simulink model "GDFLIB_FilterIIR2_BAM_F16"  (Simulink 8.3)
settings: Solver=ode45  StartTime=0.0  StopTime=10.0  RelTol=1e-3
undefined symbols (not defined in the file): f16A1, f16A2, f16B0, f16B1, f16B2
settings Model: Creator=B17364  LastModifiedBy=B17364
settings OptimizationCC: ExpressionDepthLimit=2147483647
settings DebuggingCC: FcnCallInpInsideContextMsg=UseLocalSettings  StrictBusMsg=Warning

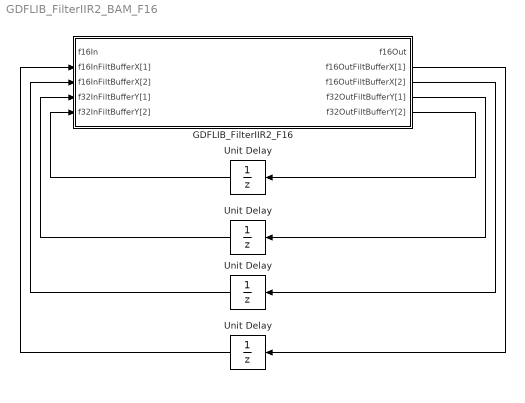
== system GDFLIB_FilterIIR2_BAM_F16 ==
  " Unit Delay" : UnitDelay  SampleTime=-1
  " Unit Delay " : UnitDelay  SampleTime=-1
  GDFLIB_FilterIIR2_F16 : Subsystem  mask(GDFLIB_FilterIIR2){f16B0=f16B0, f16B1=f16B1, f16B2=f16B2, f16A1=f16A1, f16A2=f16A2}
      mask help: Bit accurate model of direct form I second order IIR filter. All parameters as well as input and output are 16bit integers.
      mask init:
      | pos = get_param(gcb, 'Position');width = pos(3) - pos(1); height = pos(4) - pos(2);tX=width/2;tY=height*0.9;
      mask Display: color('black');port_label('input',1,'f16In');port_label('input',2,'f16InFiltBufferX[1]');port_label('input',3,'f16InFiltBufferX[2]');port_label('input',4,'f32InFiltBufferY[1]');port_label('input',5,'f32InFiltBufferY[2]');port_label('output',1,'f16Out');port_label('output',2,'f16OutFiltBufferX[1]');port_label('output',3,'f16OutFiltBufferX[2]');port_label('output',4,'f32OutFiltBufferY[1]');port_label('output',5,'f32OutFiltBufferY[2]');color('black');disp('GDFLIB_FilterIIR2_F16');color('blue');text(tX,tY, 'BAM', 'horizontalAlignment', 'center');
  Unit Delay : UnitDelay  SampleTime=-1
  "Unit Delay " : UnitDelay  SampleTime=-1
  wires:
  GDFLIB_FilterIIR2_F16/2(f16OutFiltBufferX[1]) -> " Unit Delay "/1
  GDFLIB_FilterIIR2_F16/3(f16OutFiltBufferX[2]) -> " Unit Delay"/1
  GDFLIB_FilterIIR2_F16/4(f32OutFiltBufferY[1]) -> "Unit Delay "/1
  GDFLIB_FilterIIR2_F16/5(f32OutFiltBufferY[2]) -> Unit Delay/1
  Unit Delay/1 -> GDFLIB_FilterIIR2_F16/5(f32InFiltBufferY[2])
  "Unit Delay "/1 -> GDFLIB_FilterIIR2_F16/4(f32InFiltBufferY[1])
  " Unit Delay"/1 -> GDFLIB_FilterIIR2_F16/3(f16InFiltBufferX[2])
  " Unit Delay "/1 -> GDFLIB_FilterIIR2_F16/2(f16InFiltBufferX[1])

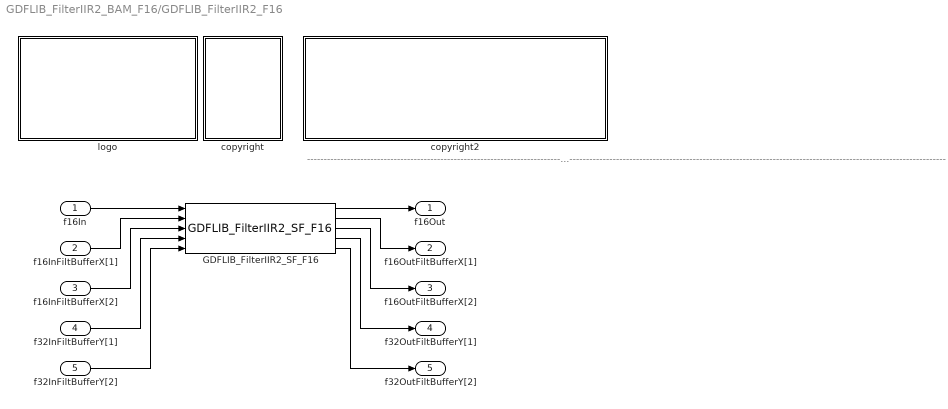
== system GDFLIB_FilterIIR2_BAM_F16/GDFLIB_FilterIIR2_F16 ==
  note: ---------------------------------------------------------------------------------------------------------------------------------------------------------------------------------------------------
  f16In : Inport
  f16InFiltBufferX[1] : Inport  Port=2
  f16InFiltBufferX[2] : Inport  Port=3
  f32InFiltBufferY[1] : Inport  Port=4
  f32InFiltBufferY[2] : Inport  Port=5
  GDFLIB_FilterIIR2_SF_F16 : S-Function  FunctionName=GDFLIB_FilterIIR2_SF_F16  Parameters=f16B0,f16B1,f16B2,f16A1,f16A2  EnableBusSupport=off
  copyright : Subsystem
      mask Display:
      | text(10,90,'FILE:');text(10,75,'DESRIPTION:')
      | text(10,60,'COPYRIGHT:')
      | text(10,45,'VERSION:')
      | text(10,30,'DATE:')
      | text(10,15,'AUTHOR:')
  copyright2 : Subsystem
      mask Display:
      | text(10,90,'GDFLIB_FilterIIR2_BAM_F16.mdl');text(10,75,'Direct form I first order IIR filter.');text(10,60,'Freescale')
      | text(10,45,'0.1');text(10,30,'08-Apr-2014');text(10,15,'');
  logo : Subsystem
      mask Display: image(imread('logo.jpg'))
  f16Out : Outport
  f16OutFiltBufferX[1] : Outport  Port=2
  f16OutFiltBufferX[2] : Outport  Port=3
  f32OutFiltBufferY[1] : Outport  Port=4
  f32OutFiltBufferY[2] : Outport  Port=5
  wires:
  f16In/1 -> GDFLIB_FilterIIR2_SF_F16/1
  GDFLIB_FilterIIR2_SF_F16/1 -> f16Out/1
  GDFLIB_FilterIIR2_SF_F16/2 -> f16OutFiltBufferX[1]/1
  GDFLIB_FilterIIR2_SF_F16/3 -> f16OutFiltBufferX[2]/1
  GDFLIB_FilterIIR2_SF_F16/5 -> f32OutFiltBufferY[2]/1
  GDFLIB_FilterIIR2_SF_F16/4 -> f32OutFiltBufferY[1]/1
  f16InFiltBufferX[1]/1 -> GDFLIB_FilterIIR2_SF_F16/2
  f16InFiltBufferX[2]/1 -> GDFLIB_FilterIIR2_SF_F16/3
  f32InFiltBufferY[1]/1 -> GDFLIB_FilterIIR2_SF_F16/4
  f32InFiltBufferY[2]/1 -> GDFLIB_FilterIIR2_SF_F16/5

== system GDFLIB_FilterIIR2_BAM_F16/GDFLIB_FilterIIR2_F16/copyright ==

== system GDFLIB_FilterIIR2_BAM_F16/GDFLIB_FilterIIR2_F16/copyright2 ==

== system GDFLIB_FilterIIR2_BAM_F16/GDFLIB_FilterIIR2_F16/logo ==
